simulink model "UK_UD"  (Simulink 8.7)
settings: Solver=VariableStepAuto  SolverMode=SingleTasking  StartTime=0  StopTime=250  FixedStep=1  RelTol=1e-3  AbsTol=1e6
libraries: dspswit3 x10, KP x8, commchan3 x1
settings Model: Creator=KDFX Team  LastModifiedBy=KDFX Team
settings DataIOCC: SignalLoggingSaveFormat=ModelDataLogs  SignalLoggingName=sigsOut
settings OptimizationCC: BooleanDataType=off
settings DebuggingCC: SaveWithParameterizedLinksMsg=none  SignalResolutionControl=TryResolveAllWithWarning  MultiTaskDSMMsg=warning  MultiTaskCondExecSysMsg=none
settings HardwareCC: TargetBitPerPointer=64  TargetLongLongMode=on  TargetIntDivRoundTo=Zero  TargetEndianess=LittleEndian  TargetWordSize=64  TargetHWDeviceType=MATLAB Host  ProdEqTarget=off
settings GRTTargetCC: GeneratePreprocessorConditionals=Use local settings  CombineOutputUpdateFcns=off  GRTInterface=on

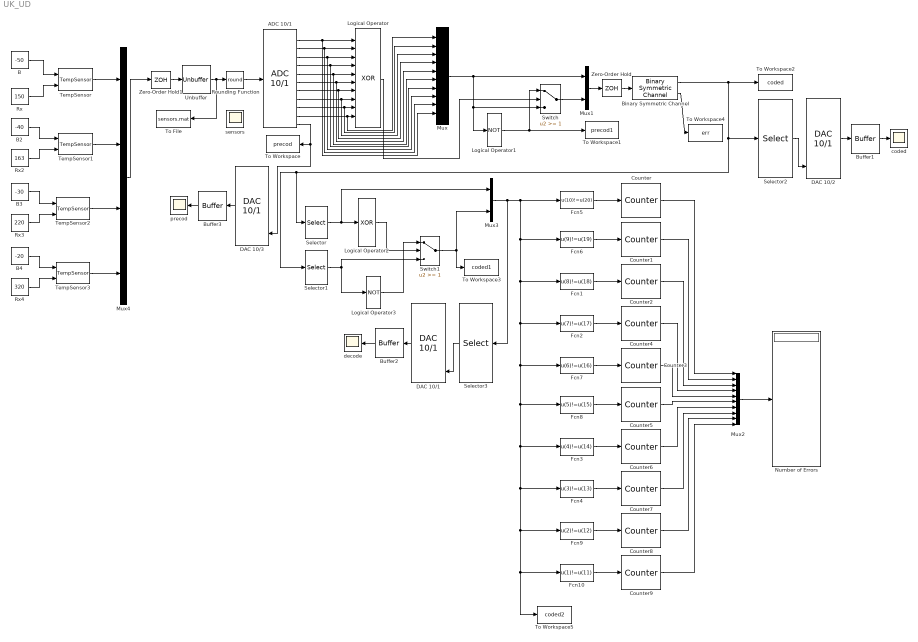
== system UK_UD ==
  ADC 10/1 : KP/ADC 10//1
  B : Constant  Value=-50
  B2 : Constant  Value=-40  SampleTime=0
  B3 : Constant  Value=-30  SampleTime=0
  B4 : Constant  Value=-20  SampleTime=0
  Binary Symmetric Channel : commchan3/Binary Symmetric Channel  P=0.06  s=2137  E=on  outDtype=double
  Buffer1 : Buffer  N=4  TreatMby1Signals=One channel  OutputFrames=off
  Buffer2 : Buffer  N=4  TreatMby1Signals=One channel  OutputFrames=off
  Buffer3 : Buffer  N=4  TreatMby1Signals=One channel  OutputFrames=off
  Counter{,1..9} (10 alike) : dspswit3/Counter  Direction=Up  CountEvent=Non-zero sample  CounterSize=User defined  MaxCount=255  InitialCount=0  Output=Count  HitValue=32  ResetInput=off  SamplesPerFrame=1  Ts=1  CntDtype=double  HitDtype=Logical
  DAC 10/1 : KP/DAC 10//1
  DAC 10/2 : KP/DAC 10//1
  DAC 10/3 : KP/DAC 10//1
  Fcn1 : Fcn  Expr=u(8)!=u(18)
  Fcn10 : Fcn  Expr=u(1)!=u(11)
  Fcn2 : Fcn  Expr=u(7)!=u(17)
  Fcn3 : Fcn  Expr=u(4)!=u(14)
  Fcn4 : Fcn  Expr=u(3)!=u(13)
  Fcn5 : Fcn  Expr=u(10)!=u(20)
  Fcn6 : Fcn  Expr=u(9)!=u(19)
  Fcn7 : Fcn  Expr=u(6)!=u(16)
  Fcn8 : Fcn  Expr=u(5)!=u(15)
  Fcn9 : Fcn  Expr=u(2)!=u(12)
  Logical Operator : Logic  Operator=XOR  Inputs=10
  Logical Operator1 : Logic  Operator=NOT  Inputs=4
  Logical Operator2 : Logic  Operator=XOR  Inputs=1
  Logical Operator3 : Logic  Operator=NOT  Inputs=4
  Mux : Mux  Inputs=10
  Mux1 : Mux  Inputs=2
  Mux2 : Mux  Inputs=10
  Mux3 : Mux  Inputs=2
  Mux4 : Mux
  Number of Errors : Display
  Rounding Function : Rounding  Operator=round
  Rx : Constant  Value=150
  Rx2 : Constant  Value=163  SampleTime=0
  Rx3 : Constant  Value=220  SampleTime=0
  Rx4 : Constant  Value=320  SampleTime=0
  Selector : Selector  InputPortWidth=20  IndexOptions=Index vector (dialog)  Indices=[1 2 3 4 5 6 7 8 9 10]  OutputSizes=1
  Selector1 : Selector  InputPortWidth=20  IndexOptions=Index vector (dialog)  Indices=[11 12 13 14 15 16 17 18 19 20]  OutputSizes=1
  Selector2 : Selector  InputPortWidth=20  IndexOptions=Index vector (dialog)  Indices=[1 2 3 4 5 6 7 8 9 10]  OutputSizes=1
  Selector3 : Selector  InputPortWidth=20  IndexOptions=Index vector (dialog)  Indices=[1 2 3 4 5 6 7 8 9 10]  OutputSizes=1
  Switch : Switch  Threshold=1  SaturateOnIntegerOverflow=on  InputSameDT=on
  Switch1 : Switch  Threshold=1  SaturateOnIntegerOverflow=on  InputSameDT=on
  TempSensor : KP/TempSensor
  TempSensor1 : KP/TempSensor
      link override Gain: Gain=0.813
  TempSensor2 : KP/TempSensor
      link override Gain: Gain=0.807
  TempSensor3 : KP/TempSensor
      link override Gain: Gain=0.835
  To File : ToFile  Filename=sensors.mat
  To Workspace : ToWorkspace  VariableName=precod  SampleTime=-1
  To Workspace1 : ToWorkspace  VariableName=precod1  SampleTime=-1
  To Workspace2 : ToWorkspace  VariableName=coded  SampleTime=-1
  To Workspace3 : ToWorkspace  VariableName=coded1  SampleTime=-1
  To Workspace4 : ToWorkspace  VariableName=err  SampleTime=-1
  To Workspace5 : ToWorkspace  VariableName=coded2  SampleTime=-1
  Unbuffer : Unbuffer  ic=4  SampleBasedProcessing=Same as frame based
  Zero-Order Hold : ZeroOrderHold
  Zero-Order Hold1 : ZeroOrderHold
  coded : Scope
  decode : Scope
  precod : Scope
  sensors : Scope
  wires:
  B/1 -> TempSensor/1
  Rx/1 -> TempSensor/2
  Rounding Function/1 -> ADC 10/1/1
  Selector/1 -> Logical Operator2/1, Mux3/1
  Logical Operator2/1 -> Switch1/2
  Selector1/1 -> Logical Operator3/1, Switch1/3
  Switch1/1 -> To Workspace3/1, Mux3/2
  Logical Operator3/1 -> Switch1/1
  Fcn2/1 -> Counter4/1
  Mux3/1 -> Selector3/1, Fcn5/1, Fcn6/1, Fcn1/1, Fcn2/1, Fcn7/1, Fcn8/1, Fcn3/1, Fcn4/1, Fcn9/1, To Workspace5/1, Fcn10/1
  Fcn1/1 -> Counter2/1
  Fcn5/1 -> Counter/1
  Fcn6/1 -> Counter1/1
  Binary Symmetric Channel/2 -> To Workspace4/1
  ADC 10/1/2 -> Logical Operator/1, Mux/10
  ADC 10/1/3 -> Logical Operator/2, Mux/9
  ADC 10/1/4 -> Logical Operator/3, Mux/8
  ADC 10/1/5 -> Logical Operator/4, Mux/7
  ADC 10/1/6 -> Logical Operator/5, Mux/6
  ADC 10/1/7 -> Logical Operator/6, Mux/5
  ADC 10/1/8 -> Logical Operator/7, Mux/4
  ADC 10/1/9 -> Logical Operator/8, Mux/3
  ADC 10/1/10 -> Logical Operator/9, Mux/2
  ADC 10/1/11 -> Logical Operator/10, Mux/1
  ADC 10/1/12 -> DAC 10/3/11, To Workspace/1
  Logical Operator/1 -> Switch/2
  Logical Operator1/1 -> Switch/1, To Workspace1/1
  Switch/1 -> Mux1/2
  Mux1/1 -> Zero-Order Hold/1
  Mux/1 -> Logical Operator1/1, Switch/3, Mux1/1
  Fcn4/1 -> Counter7/1
  Fcn3/1 -> Counter6/1
  Fcn7/1 -> Counter3/1
  Fcn8/1 -> Counter5/1
  Fcn10/1 -> Counter9/1
  Counter/1 -> Mux2/1
  Counter1/1 -> Mux2/2
  Counter2/1 -> Mux2/3
  Counter4/1 -> Mux2/4
  Counter3/1 -> Mux2/5
  Counter9/1 -> Mux2/10
  Counter8/1 -> Mux2/9
  Counter7/1 -> Mux2/8
  Counter6/1 -> Mux2/7
  Counter5/1 -> Mux2/6
  Fcn9/1 -> Counter8/1
  Zero-Order Hold/1 -> Binary Symmetric Channel/1
  B2/1 -> TempSensor1/1
  Rx2/1 -> TempSensor1/2
  B3/1 -> TempSensor2/1
  Rx3/1 -> TempSensor2/2
  B4/1 -> TempSensor3/1
  Rx4/1 -> TempSensor3/2
  Zero-Order Hold1/1 -> Unbuffer/1
  Mux4/1 -> Zero-Order Hold1/1
  TempSensor/1 -> Mux4/1
  TempSensor1/1 -> Mux4/2
  TempSensor2/1 -> Mux4/3
  TempSensor3/1 -> Mux4/4
  Mux2/1 -> Number of Errors/1
  Binary Symmetric Channel/1 -> To Workspace2/1, Selector2/1, Selector/1, Selector1/1
  Selector3/1 -> DAC 10/1/11
  DAC 10/1/1 -> Buffer2/1
  Buffer2/1 -> decode/1
  Buffer1/1 -> coded/1
  Selector2/1 -> DAC 10/2/11
  DAC 10/2/1 -> Buffer1/1
  Buffer3/1 -> precod/1
  DAC 10/3/1 -> Buffer3/1
  Unbuffer/1 -> To File/1, Rounding Function/1
